simulink model "Tuned_like_Lag"  (R2020b)
settings: Solver=VariableStepAuto  StartTime=0.0  StopTime=3  RelTol=1e-3
libraries: pid_lib x2
settings Model: Creator=barak  LastModifiedBy=barak
settings DataIOCC: ReturnWorkspaceOutputs=off
settings DebuggingCC: ArithmeticOperatorsInVariantConditions=warning
settings SFSimCC: SimUseLocalCustomCode=off  CustomCodeUndefinedFunction=UseInterfaceOnly
settings RTWCC: RTWUseLocalCustomCode=off

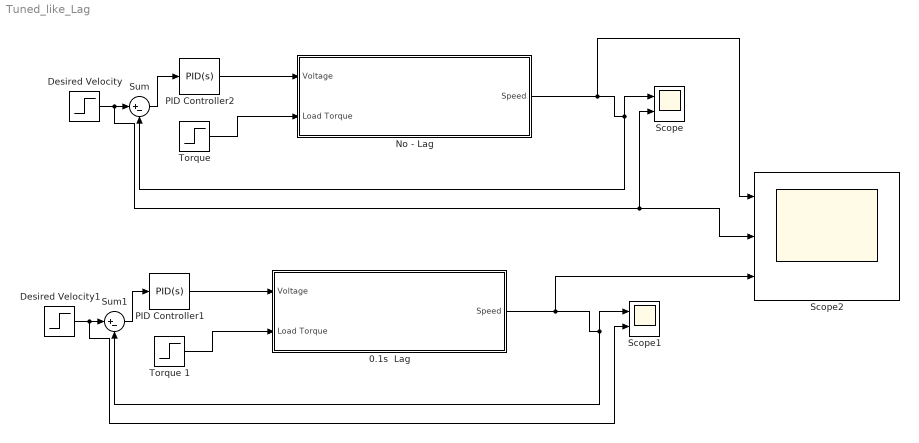
== system Tuned_like_Lag ==
  0.1s  Lag : Subsystem
  Desired Velocity : Step  After=10  SampleTime=0
  Desired Velocity1 : Step  After=10  SampleTime=0
  No - Lag : Subsystem
  PID Controller1 : pid_lib/PID Controller  Controller=PID  Form=Parallel  TimeDomain=Continuous-time  UseExternalTs=off  SampleTime=-1  IntegratorMethod=Forward Euler  FilterMethod=Forward Euler  ControllerParametersSource=internal  P=0.136705612158136  I=1.99708162581554  D=-0.00342604783089772  UseFilter=on  N=8.28752680701693  TunerSelectOption=Transfer Function Based (PID Tuner App)  InitialConditionSource=internal  InitialConditionForIntegrator=0  InitialConditionForFilter=0  DifferentiatorICPrevScaledInput=0  ExternalReset=none  TrackingMode=off  Kt=1  LimitOutput=off  SatLimitsSource=internal  UpperSaturationLimit=inf  LowerSaturationLimit=-inf  LinearizeAsGain=on  AntiWindupMode=none  Kb=1  POutMin=[]  POutMax=[]  IOutMin=[]  IOutMax=[]  DOutMin=[]  DOutMax=[]  NOutMin=[]  NOutMax=[]  SumOutMin=[]  SumOutMax=[]  SaturationOutMin=[]  SaturationOutMax=[]  PParamMin=[]  PParamMax=[]  IParamMin=[]  IParamMax=[]  DParamMin=[]  DParamMax=[]  NParamMin=[]  NParamMax=[]  KbParamMin=[]  KbParamMax=[]  KtParamMin=[]  KtParamMax=[]  KbOutMin=[]  KbOutMax=[]  KtOutMin=[]  KtOutMax=[]  IntegratorOutMin=[]  IntegratorOutMax=[]  FilterOutMin=[]  FilterOutMax=[]  SumI1OutMin=[]  SumI1OutMax=[]  SumI2OutMin=[]  SumI2OutMax=[]  SumI3OutMin=[]  SumI3OutMax=[]  SumI4OutMin=[]  SumI4OutMax=[]  SumDOutMin=[]  SumDOutMax=[]  DifferentiatorOutMin=[]  DifferentiatorOutMax=[]  FilterDiffOutCoefMin=[]  FilterDiffOutCoefMax=[]  ReciprocalOutMin=[]  ReciprocalOutMax=[]  SumDenOutMin=[]  SumDenOutMax=[]  SumNumOutMin=[]  SumNumOutMax=[]  DivideOutMin=[]  DivideOutMax=[]  UdiffTsProdOutMin=[]  UdiffTsProdOutMax=[]  NTsProdOutMin=[]  NTsProdOutMax=[]  UintegralTsProdOutMin=[]  UintegralTsProdOutMax=[]  UngainTsProdOutMin=[]  UngainTsProdOutMax=[]  IntegratorContinuousStateAttributes=''  IntegratorStateMustResolveToSignalObject=off  IntegratorRTWStateStorageClass=Auto  FilterContinuousStateAttributes=''  FilterStateMustResolveToSignalObject=off  FilterRTWStateStorageClass=Auto  ParallelPVariant=InternalParameters  IdealPVariant=Disabled  IVariant=InternalParameters  DVariant=InternalParameters  IntegratorVariant=Continuous  SatVariant=Disabled  AWVariant=Passthrough  PCopyVariant=Disabled  TRVariant=Disabled  FdbkBlocksVariant=Forward  IdealPFdbkVariant=Disabled  SatFdbkVariant=Disabled  DerivativeFilterVariant=ContFilter  NVariant=InternalParameters  NCopyVariant=Disabled  FilterICVariant=InternalICsFilter  IntegratorICVariant=InternalICs  ExternalResetVariant=Disabled  TRSumVariant=Passthrough  SumFdbkVariant=Disabled  SumVariant=Sum_PID  TsampFilterVariant=InternalTs  TsampNgainVariant=Passthrough  TsampIntegralVariant=Passthrough  ExternalSaturationOutDataTypeStr=Inherit: Same as second input
  PID Controller2 : pid_lib/PID Controller  Controller=PID  Form=Parallel  TimeDomain=Continuous-time  UseExternalTs=off  SampleTime=-1  IntegratorMethod=Forward Euler  FilterMethod=Forward Euler  ControllerParametersSource=internal  P=0.136705612158136  I=1.99708162581554  D=-0.00342604783089772  UseFilter=on  N=8.28752680701693  TunerSelectOption=Transfer Function Based (PID Tuner App)  InitialConditionSource=internal  InitialConditionForIntegrator=0  InitialConditionForFilter=0  DifferentiatorICPrevScaledInput=0  ExternalReset=none  TrackingMode=off  Kt=1  LimitOutput=off  SatLimitsSource=internal  UpperSaturationLimit=inf  LowerSaturationLimit=-inf  LinearizeAsGain=on  AntiWindupMode=none  Kb=1  POutMin=[]  POutMax=[]  IOutMin=[]  IOutMax=[]  DOutMin=[]  DOutMax=[]  NOutMin=[]  NOutMax=[]  SumOutMin=[]  SumOutMax=[]  SaturationOutMin=[]  SaturationOutMax=[]  PParamMin=[]  PParamMax=[]  IParamMin=[]  IParamMax=[]  DParamMin=[]  DParamMax=[]  NParamMin=[]  NParamMax=[]  KbParamMin=[]  KbParamMax=[]  KtParamMin=[]  KtParamMax=[]  KbOutMin=[]  KbOutMax=[]  KtOutMin=[]  KtOutMax=[]  IntegratorOutMin=[]  IntegratorOutMax=[]  FilterOutMin=[]  FilterOutMax=[]  SumI1OutMin=[]  SumI1OutMax=[]  SumI2OutMin=[]  SumI2OutMax=[]  SumI3OutMin=[]  SumI3OutMax=[]  SumI4OutMin=[]  SumI4OutMax=[]  SumDOutMin=[]  SumDOutMax=[]  DifferentiatorOutMin=[]  DifferentiatorOutMax=[]  FilterDiffOutCoefMin=[]  FilterDiffOutCoefMax=[]  ReciprocalOutMin=[]  ReciprocalOutMax=[]  SumDenOutMin=[]  SumDenOutMax=[]  SumNumOutMin=[]  SumNumOutMax=[]  DivideOutMin=[]  DivideOutMax=[]  UdiffTsProdOutMin=[]  UdiffTsProdOutMax=[]  NTsProdOutMin=[]  NTsProdOutMax=[]  UintegralTsProdOutMin=[]  UintegralTsProdOutMax=[]  UngainTsProdOutMin=[]  UngainTsProdOutMax=[]  IntegratorContinuousStateAttributes=''  IntegratorStateMustResolveToSignalObject=off  IntegratorRTWStateStorageClass=Auto  FilterContinuousStateAttributes=''  FilterStateMustResolveToSignalObject=off  FilterRTWStateStorageClass=Auto  ParallelPVariant=InternalParameters  IdealPVariant=Disabled  IVariant=InternalParameters  DVariant=InternalParameters  IntegratorVariant=Continuous  SatVariant=Disabled  AWVariant=Passthrough  PCopyVariant=Disabled  TRVariant=Disabled  FdbkBlocksVariant=Forward  IdealPFdbkVariant=Disabled  SatFdbkVariant=Disabled  DerivativeFilterVariant=ContFilter  NVariant=InternalParameters  NCopyVariant=Disabled  FilterICVariant=InternalICsFilter  IntegratorICVariant=InternalICs  ExternalResetVariant=Disabled  TRSumVariant=Passthrough  SumFdbkVariant=Disabled  SumVariant=Sum_PID  TsampFilterVariant=InternalTs  TsampNgainVariant=Passthrough  TsampIntegralVariant=Passthrough  ExternalSaturationOutDataTypeStr=Inherit: Same as second input
  Scope : Scope  NumInputPorts=2
  Scope1 : Scope  NumInputPorts=2
  Scope2 : Scope  NumInputPorts=3
  Sum : Sum  Inputs=|+-
  Sum1 : Sum  Inputs=|+-
  "Torque " : Step  Time=20  After=0  SampleTime=0
  Torque 1 : Step  Time=20  After=0  SampleTime=0
  wires:
  PID Controller2/1 -> No - Lag/1(Voltage)
  Sum/1 -> PID Controller2/1
  "Torque "/1 -> No - Lag/2("Load Torque ")
  No - Lag/1("Speed ") -> Scope2/1, Scope/1, Sum/2
  PID Controller1/1 -> 0.1s  Lag/1(Voltage)
  Desired Velocity1/1 -> Scope1/2, Sum1/1
  Torque 1/1 -> 0.1s  Lag/2("Load Torque ")
  Sum1/1 -> PID Controller1/1
  0.1s  Lag/1("Speed ") -> Scope2/3, Scope1/1, Sum1/2
  Desired Velocity/1 -> Scope2/2, Scope/2, Sum/1

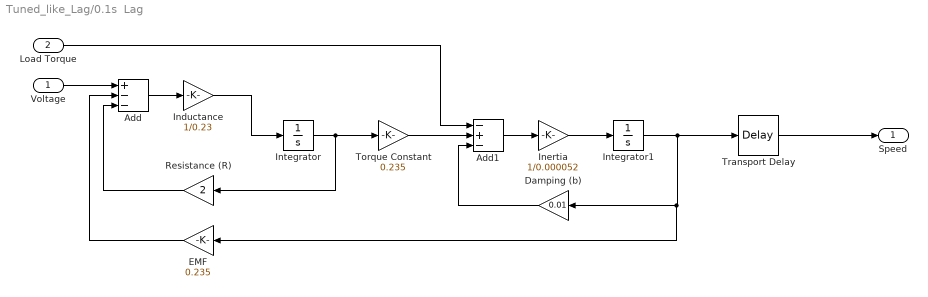
== system Tuned_like_Lag/0.1s  Lag ==
  Voltage : Inport
  "Load Torque " : Inport  Port=2
  Add : Sum  Inputs=+--
  Add1 : Sum  Inputs=-+-
  Damping (b) : Gain  Gain=0.01
  EMF : Gain  Gain=0.235
  Inductance : Gain  Gain=1/0.23
  "Inertia " : Gain  Gain=1/0.000052
  Integrator : Integrator
  Integrator1 : Integrator
  Resistance (R) : Gain  Gain=2
  Torque Constant : Gain  Gain=0.235
  Transport Delay : TransportDelay  DelayTime=0.1
  "Speed " : Outport  VectorParamsAs1DForOutWhenUnconnected=off
  wires:
  Voltage/1 -> Add/1
  Add/1 -> Inductance/1
  Inductance/1 -> Integrator/1
  Integrator/1 -> Resistance (R)/1, Torque Constant/1
  Resistance (R)/1 -> Add/3
  Add1/1 -> "Inertia "/1
  "Inertia "/1 -> Integrator1/1
  EMF/1 -> Add/2
  "Load Torque "/1 -> Add1/1
  Torque Constant/1 -> Add1/2
  Damping (b)/1 -> Add1/3
  Integrator1/1 -> Transport Delay/1, EMF/1, Damping (b)/1
  Transport Delay/1 -> "Speed "/1

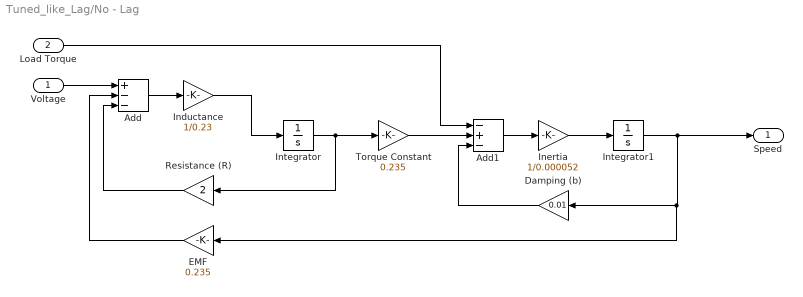
== system Tuned_like_Lag/No - Lag ==
  Voltage : Inport
  "Load Torque " : Inport  Port=2
  Add : Sum  Inputs=+--
  Add1 : Sum  Inputs=-+-
  Damping (b) : Gain  Gain=0.01
  EMF : Gain  Gain=0.235
  Inductance : Gain  Gain=1/0.23
  "Inertia " : Gain  Gain=1/0.000052
  Integrator : Integrator
  Integrator1 : Integrator
  Resistance (R) : Gain  Gain=2
  Torque Constant : Gain  Gain=0.235
  "Speed " : Outport  VectorParamsAs1DForOutWhenUnconnected=off
  wires:
  Voltage/1 -> Add/1
  Add/1 -> Inductance/1
  Inductance/1 -> Integrator/1
  Integrator/1 -> Resistance (R)/1, Torque Constant/1
  Resistance (R)/1 -> Add/3
  Add1/1 -> "Inertia "/1
  "Inertia "/1 -> Integrator1/1
  EMF/1 -> Add/2
  "Load Torque "/1 -> Add1/1
  Torque Constant/1 -> Add1/2
  Damping (b)/1 -> Add1/3
  Integrator1/1 -> "Speed "/1, EMF/1, Damping (b)/1
